simulink model "BD_PAR_AUTO"  (Simulink 7.9)
settings: Solver=ode1  SolverMode=SingleTasking  StartTime=0.0  StopTime=max(cyc_mph(:,1))  FixedStep=1  MaxStep=1  RelTol=1e-3  AbsTol=1e-3
undefined symbols (not defined in the file): ess_on, ex_calc, fc_emis, fc_max_trq, fc_trq_scale, vc_idle_spd
libraries: lib_transmission x5, lib_wheel x2, lib_controls x2, lib_help x2, lib_accessory x2, lib_outputs x1, lib_interactive x1, lib_drive_cycle x1, lib_energy_storage x1, lib_exhaust x1, lib_fuel_converter x1, lib_electric_machine x1
settings Model: Creator=mokeefe  LastModifiedBy=mokeefe  ExtModeTrigMode=oneshot  ExtModeArmWhenConnect=off
settings Model: ModifiedComment=|
  | mokeefe -- Fri Apr 06 09:23:46 2012 -- Version 1.22
  | Restore all library links and save to latest version.
settings Model: ModifiedHistory=|
  | mokeefe -- Fri Apr 06 09:23:46 2012 -- Version 1.22
  | Restore all library links and save to latest version.
  | 
  | ssprik -- Wed Sep 24 15:05:16 2003 -- Version 1.21
  | 
  | 
  | mokeefe -- Fri Aug 30 07:45:49 2002 -- Version 1.20
  | Changed the input to "mechanical accessory loads <acc>/Mechanical Accessory Loads V2 <acc>" masked parameter input blocks. In R13, the function "not" no longer returns double 1 or double 0 for true and false but instead returns type logical (boolean). Thus, I am now multiplying by double 1 which causes a type conversion to double yielding the desired effect.
  | 
  | 
  | abrooker -- Tue May 14 11:45:21 2002 -- Version 1.19
  | 
  | 
  | mokeefe -- Thu Apr 18 08:00:10 2002 -- Version 1.18
  | saving the model:
  | o "without the model browser open"
  | o with only top-level screen visible
  | o and with "fit to view" enabled
settings DataIOCC: LimitDataPoints=off  SaveOutput=off  SaveTime=off
settings OptimizationCC: BooleanDataType=off
settings DebuggingCC: SaveWithParameterizedLinksMsg=none  SignalResolutionControl=TryResolveAllWithWarning  SolverPrmCheckMsg=none  MultiTaskDSMMsg=warning  MultiTaskCondExecSysMsg=none  UnconnectedLineMsg=none  StrictBusMsg=None
settings HardwareCC: TargetUnknown=on
settings RTWCC: TemplateMakefile=grt_vc.tmf  IncludeERTFirstTime=on
settings GRTTargetCC: CombineOutputUpdateFcns=off  GRTInterface=on

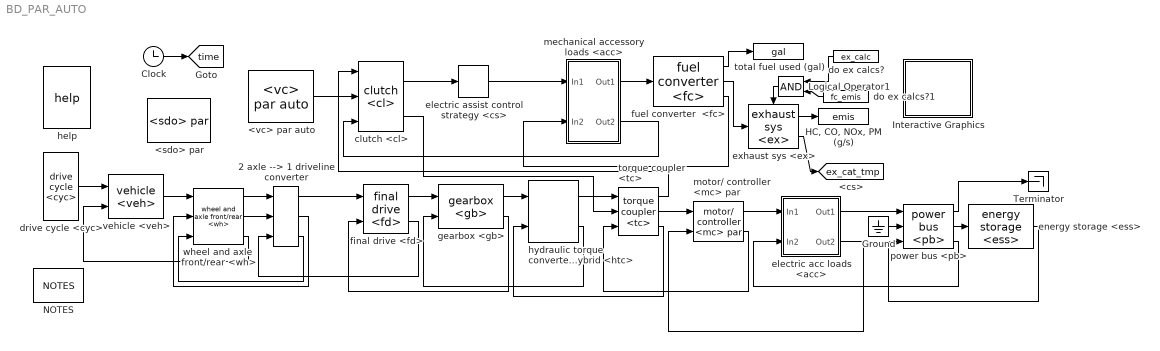
== system BD_PAR_AUTO ==
  2 axle --> 1 driveline converter : lib_wheel/2 axle --> 1 driveline converter
  <sdo> par : lib_outputs/<sdo> par  SystemSampleTime=-1
  <vc> par auto : lib_controls/<vc> par auto  SystemSampleTime=-1
  Clock : Clock
  Ground : Ground
  "HC, CO, NOx, PM (g/s)" : ToWorkspace  VariableName=emis
  Interactive Graphics : Subsystem  BlockChoice=off
      settings: AttributesFormatString=%<BlockChoice>  TemplateBlock=lib_interactive/Interactive Graphics  MemberBlocks=off,on
  Logical Operator1 : Logic
  NOTES : lib_help/NOTES  SystemSampleTime=-1
  Terminator : Terminator
  clutch <cl> : lib_transmission/clutch <cl>  slip_spd=vc_launch_spd  maxtrq=max(fc_max_trq)*fc_trq_scale
  do ex calcs? : Constant  Value=ex_calc
  do ex calcs?1 : Constant  Value=fc_emis
  drive cycle <cyc> : lib_drive_cycle/drive cycle <cyc>  SystemSampleTime=-1
  electric acc loads <acc> : Subsystem
      mask Display: image(imread('bdi_acc_elec.bmp'))
  electric assist control strategy <cs> : lib_controls/electric assist control strategy <cs>  SystemSampleTime=-1
  energy storage <ess> : lib_energy_storage/energy storage <ess>  SystemSampleTime=-1
  exhaust sys <ex> : lib_exhaust/exhaust sys <ex>  SystemSampleTime=-1
  final drive <fd> : lib_transmission/final drive <fd>  SystemSampleTime=-1
  fuel converter  <fc> : lib_fuel_converter/fuel converter  <fc>  SystemSampleTime=-1
  gearbox <gb> : lib_transmission/gearbox <gb>  SystemSampleTime=-1
  help : lib_help/help  SystemSampleTime=-1
  hydraulic torque converter for  parallel hybrid <htc> : lib_transmission/hydraulic torque converter for  parallel hybrid <htc>  SystemSampleTime=-1
  mechanical accessory loads <acc> : Subsystem
      mask Display: image(imread('bdi_acc_pic.bmp'))
  motor/ controller <mc> par : lib_electric_machine/motor// controller <mc> par  SystemSampleTime=-1
  power bus <pb> : lib_power_bus/power bus <pb>  SystemSampleTime=-1
  torque coupler <tc> : lib_transmission/torque coupler <tc>  SystemSampleTime=-1
  total fuel used (gal) : ToWorkspace  VariableName=gal
  vehicle <veh> : lib_vehicle/vehicle <veh>  SystemSampleTime=-1
  wheel and axle  front/rear <wh> : lib_wheel/wheel and axle  front//rear <wh>  SystemSampleTime=-1
  tag scope: ex_cat_tmp=global, time=global
  wires:
  vehicle <veh>/1 -> wheel and axle  front/rear <wh>/1
  wheel and axle  front/rear <wh>/3 -> vehicle <veh>/2
  2 axle --> 1 driveline converter/1 -> final drive <fd>/1
  final drive <fd>/2 -> 2 axle --> 1 driveline converter/3
  final drive <fd>/1 -> gearbox <gb>/1
  drive cycle <cyc>/1 -> vehicle <veh>/1
  clutch <cl>/1 -> electric assist control strategy <cs>/1
  fuel converter  <fc>/2 -> exhaust sys <ex>/1
  do ex calcs?/1 -> Logical Operator1/1
  fuel converter  <fc>/1 -> total fuel used (gal)/1
  exhaust sys <ex>/1 -> "HC, CO, NOx, PM (g/s)"/1
  Logical Operator1/1 -> exhaust sys <ex>/Enable
  do ex calcs?1/1 -> Logical Operator1/2
  Clock/1 -> [time]
  gearbox <gb>/2 -> final drive <fd>/2
  clutch <cl>/2 -> torque coupler <tc>/2
  <vc> par auto/1 -> clutch <cl>/2
  torque coupler <tc>/1 -> clutch <cl>/1
  motor/ controller <mc> par/2 -> torque coupler <tc>/3
  Ground/1 -> power bus <pb>/2
  power bus <pb>/2 -> energy storage <ess>/1
  power bus <pb>/1 -> Terminator/1
  energy storage <ess>/1 -> power bus <pb>/3
  torque coupler <tc>/2 -> motor/ controller <mc> par/1
  gearbox <gb>/1 -> hydraulic torque converter for  parallel hybrid <htc>/1
  hydraulic torque converter for  parallel hybrid <htc>/1 -> torque coupler <tc>/1
  hydraulic torque converter for  parallel hybrid <htc>/2 -> gearbox <gb>/2
  torque coupler <tc>/3 -> hydraulic torque converter for  parallel hybrid <htc>/2
  exhaust sys <ex>/2 -> [ex_cat_tmp]
  motor/ controller <mc> par/1 -> electric acc loads <acc>/1(In1)
  electric acc loads <acc>/1(Out1) -> power bus <pb>/1
  power bus <pb>/3 -> electric acc loads <acc>/2(In2)
  electric acc loads <acc>/2(Out2) -> motor/ controller <mc> par/2
  electric assist control strategy <cs>/1 -> mechanical accessory loads <acc>/1(In1)
  mechanical accessory loads <acc>/1(Out1) -> fuel converter  <fc>/1
  fuel converter  <fc>/3 -> mechanical accessory loads <acc>/2(In2)
  mechanical accessory loads <acc>/2(Out2) -> clutch <cl>/3
  wheel and axle  front/rear <wh>/1 -> 2 axle --> 1 driveline converter/1
  wheel and axle  front/rear <wh>/2 -> 2 axle --> 1 driveline converter/2
  2 axle --> 1 driveline converter/2 -> wheel and axle  front/rear <wh>/2
  2 axle --> 1 driveline converter/3 -> wheel and axle  front/rear <wh>/3

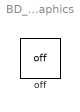
== system BD_PAR_AUTO/Interactive Graphics ==
  off : lib_interactive/off  Tag=Altia_off  SystemSampleTime=-1

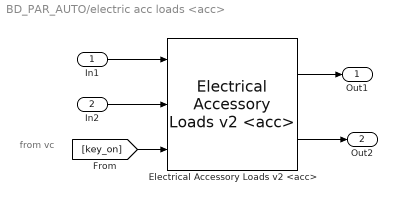
== system BD_PAR_AUTO/electric acc loads <acc> ==
  note: from vc
  In1 : Inport
  In2 : Inport  Port=2
  Electrical Accessory Loads v2 <acc> : lib_accessory/Electrical Accessory Loads v2 <acc>  load_on=ess_on
  Out1 : Outport
  Out2 : Outport  Port=2
  wires:
  In1/1 -> Electrical Accessory Loads v2 <acc>/1
  In2/1 -> Electrical Accessory Loads v2 <acc>/2
  Electrical Accessory Loads v2 <acc>/1 -> Out1/1
  Electrical Accessory Loads v2 <acc>/2 -> Out2/1
  [key_on] -> Electrical Accessory Loads v2 <acc>/3

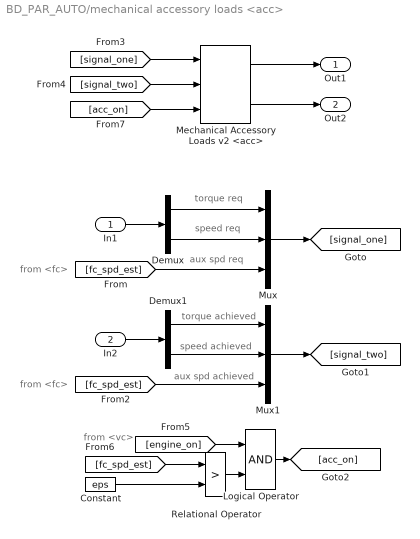
== system BD_PAR_AUTO/mechanical accessory loads <acc> ==
  note: from <fc>
  note: from <fc>
  note: torque req
  note: speed req
  note: aux spd req
  note: torque achieved
  note: speed achieved
  note: aux spd achieved
  note: from <vc>
  In1 : Inport
  In2 : Inport  Port=2
  Constant : Constant  Value=eps
  Demux : Demux  Outputs=2
  Demux1 : Demux  Outputs=2
  Logical Operator : Logic
  Mechanical Accessory Loads v2 <acc> : lib_accessory/Mechanical Accessory Loads v2 <acc>  load_on=not(ess_on)*1  acc_max_spd=inf  acc_min_spd=vc_idle_spd+eps  ic_mech_trq=0  ic_mech_pwr=0
  Mux : Mux  Inputs=3
  Mux1 : Mux  Inputs=3
  Relational Operator : RelationalOperator  Operator=>  InputSameDT=on
  Out1 : Outport
  Out2 : Outport  Port=2
  wires:
  [signal_one] -> Mechanical Accessory Loads v2 <acc>/1
  Mechanical Accessory Loads v2 <acc>/1 -> Out1/1
  Mechanical Accessory Loads v2 <acc>/2 -> Out2/1
  [signal_two] -> Mechanical Accessory Loads v2 <acc>/2
  [acc_on] -> Mechanical Accessory Loads v2 <acc>/3
  Mux/1 -> [signal_one]
  In1/1 -> Demux/1
  Demux/1 -> Mux/1
  Demux/2 -> Mux/2
  [fc_spd_est] -> Mux/3
  Mux1/1 -> [signal_two]
  In2/1 -> Demux1/1
  Demux1/1 -> Mux1/1
  Demux1/2 -> Mux1/2
  [fc_spd_est] -> Mux1/3
  [fc_spd_est] -> Relational Operator/1
  Constant/1 -> Relational Operator/2
  [engine_on] -> Logical Operator/1
  Relational Operator/1 -> Logical Operator/2
  Logical Operator/1 -> [acc_on]
